simulink model "linear_model"  (Simulink 5.0)
settings: Solver=ode45  StartTime=0.0  StopTime=0.01  FixedStep=0.0001  RelTol=1e-3
libraries: simulink x1
settings Model: LastModifiedBy=Oracle  OptimizeBlockIOStorage=off  RTWOptions="-aEnforceIntegerDowncast=1 -aExtMode=0 -aExtModeTesting=0 -aFoldNonRolledExpr=1 -aForceParamTrailComments=0 -aGenerateComments=1 -aGenerateReport=0 -aIgnoreCustomStorageClasses=1 -aIncDataTypeInIds=0 -aIncHierarchyInIds=0 -aInlineInvariantSignals=1 -aInlineParameters=0 -aInlinedPrmAccess=\"Literals\" -aLocalBlockOutputs=1 -aLogVarNameModifier=\"rt_\" -aMaxRTWIdLen=31 -aPrefixModelToSubsysFcnNames=1 -aRTWVerbose=1 -aRollThreshold=5 -aShowEliminatedStatements=0"

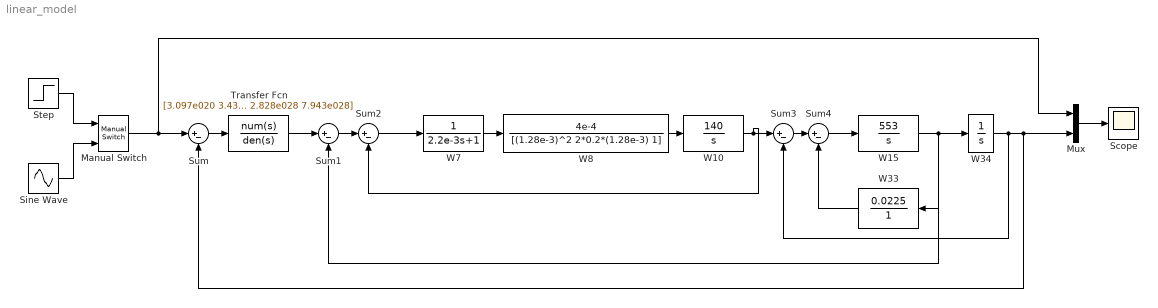
== system linear_model ==
  Manual Switch : simulink/Signal Routing/Manual Switch  sw=0  action=0
  Mux : Mux  Inputs=2
  Scope : Scope
      settings: TimeRange=5  YMin=0  YMax=1
  Sine Wave : Sin  Frequency=1200  SampleTime=0
  Step : Step  Time=0  SampleTime=0
  Sum{,1..4} (5 alike) : Sum  Inputs=|+-  SaturateOnIntegerOverflow=on
  Transfer Fcn : TransferFcn  Numerator=[3.097e020 3.437e023 3.251e026 1.485e029 1.737e031 2.722e032 8.528e033 9.532e032 ]  Denominator=[1 1.539e006 8.565e011 2.152e017 2.439e022 1.001e027 2.828e028 7.943e028]
  W10 : TransferFcn  Numerator=[140]  Denominator=[1 0]
  W15 : TransferFcn  Numerator=[553]  Denominator=[1 0]
  W33 : TransferFcn  Orientation=left  Numerator=[0.0225]  Denominator=[1]
  W34 : TransferFcn  Denominator=[1 0]
  W7 : TransferFcn  Denominator=[2.2e-3 1]
  W8 : TransferFcn  Numerator=[4e-4]  Denominator=[(1.28e-3)^2 2*0.2*(1.28e-3) 1]
  wires:
  Sum2/1 -> W7/1
  W7/1 -> W8/1
  W8/1 -> W10/1
  W10/1 -> Sum3/1, Sum2/2
  Sum3/1 -> Sum4/1
  Sum4/1 -> W15/1
  W15/1 -> Sum1/2, W34/1, W33/1
  Step/1 -> Manual Switch/1
  Sine Wave/1 -> Manual Switch/2
  Mux/1 -> Scope/1
  Manual Switch/1 -> Mux/1, Sum/1
  Sum1/1 -> Sum2/1
  Sum/1 -> Transfer Fcn/1
  W34/1 -> Sum3/2, Sum/2, Mux/2
  W33/1 -> Sum4/2
  Transfer Fcn/1 -> Sum1/1
